simulink model "case2"  (R2024b)
settings: Solver=FixedStepAuto  StartTime=0  StopTime=1  FixedStep=1e-7  RelTol=1e-3
values from neighbouring files (symbols this model uses):
  SG_D_1_D = 0.01056    [IEEE9_case_parameters.m]    (also in case1_parameters.m; case2_parameters.m; case3_parameters.m; case4_parameters.m)
  SG_D_1_EnableSaturation = 0    [IEEE9_case_parameters.m]    (also in case1_parameters.m; case2_parameters.m; case3_parameters.m; case4_parameters.m)
  SG_D_1_f0 = 60    [IEEE9_case_parameters.m]    (also in case1_parameters.m; case2_parameters.m; case3_parameters.m; case4_parameters.m)
  SG_D_1_H = 7.5    [IEEE9_case_parameters.m]    (also in case1_parameters.m; case2_parameters.m; case3_parameters.m; case4_parameters.m)
  SG_D_1_K_A = 20    [IEEE9_case_parameters.m]    (also in case1_parameters.m; case2_parameters.m; case3_parameters.m; case4_parameters.m)
  SG_D_1_K_E = 1.000000e+1    (= 10)    [IEEE9_case_parameters.m]    (also in case1_parameters.m; case2_parameters.m; case3_parameters.m; case4_parameters.m)
  SG_D_1_K_F = 2.363    [IEEE9_case_parameters.m]    (also in case1_parameters.m; case2_parameters.m; case3_parameters.m; case4_parameters.m)
  SG_D_1_K_s = 0.5    [IEEE9_case_parameters.m]    (also in case1_parameters.m = 5; case2_parameters.m = 5; case3_parameters.m = 5; case4_parameters.m = 5)
  SG_D_1_R_a = 0.001088    [IEEE9_case_parameters.m]    (also in case1_parameters.m; case2_parameters.m; case3_parameters.m; case4_parameters.m)
  SG_D_1_S_A = 1    [IEEE9_case_parameters.m]    (also in case1_parameters.m; case2_parameters.m; case3_parameters.m; case4_parameters.m)
  SG_D_1_S_B = 0.103    [IEEE9_case_parameters.m]    (also in case1_parameters.m; case2_parameters.m; case3_parameters.m; case4_parameters.m)
  SG_D_1_S_N = 10.659857    [IEEE9_case_parameters.m]    (also in case1_parameters.m; case2_parameters.m; case3_parameters.m; case4_parameters.m)
  SG_D_1_SpeedPara = 200    [IEEE9_case_parameters.m]    (also in case1_parameters.m; case2_parameters.m; case3_parameters.m; case4_parameters.m)
  SG_D_1_T_0 = 0.720173    [IEEE9_case_parameters.m]    (also in case1_parameters.m = 0.755522; case2_parameters.m = 0.808931; case3_parameters.m = 0.869402; case4_parameters.m = 0.729316)
  SG_D_1_T_1 = 0.3    [IEEE9_case_parameters.m]    (also in case1_parameters.m; case2_parameters.m; case3_parameters.m; case4_parameters.m)
  SG_D_1_T_2 = 0.05    [IEEE9_case_parameters.m]    (also in case1_parameters.m; case2_parameters.m; case3_parameters.m; case4_parameters.m)
  SG_D_1_T_3 = 0.02    [IEEE9_case_parameters.m]    (also in case1_parameters.m; case2_parameters.m; case3_parameters.m; case4_parameters.m)
  SG_D_1_T_4 = 0.005    [IEEE9_case_parameters.m]    (also in case1_parameters.m; case2_parameters.m; case3_parameters.m; case4_parameters.m)
  SG_D_1_T_A = 0.02    [IEEE9_case_parameters.m]    (also in case1_parameters.m; case2_parameters.m; case3_parameters.m; case4_parameters.m)
  SG_D_1_T_dd = 8.000000e+0    (= 8)    [IEEE9_case_parameters.m]    (also in case1_parameters.m; case2_parameters.m; case3_parameters.m; case4_parameters.m)
  SG_D_1_T_ddd = 0.04    [IEEE9_case_parameters.m]    (also in case1_parameters.m; case2_parameters.m; case3_parameters.m; case4_parameters.m)
  SG_D_1_T_E = 0.314    [IEEE9_case_parameters.m]    (also in case1_parameters.m; case2_parameters.m; case3_parameters.m; case4_parameters.m)
  SG_D_1_T_F = 0.35    [IEEE9_case_parameters.m]    (also in case1_parameters.m; case2_parameters.m; case3_parameters.m; case4_parameters.m)
  SG_D_1_T_qd = 0.8    [IEEE9_case_parameters.m]    (also in case1_parameters.m; case2_parameters.m; case3_parameters.m; case4_parameters.m)
  SG_D_1_T_qdd = 0.02    [IEEE9_case_parameters.m]    (also in case1_parameters.m; case2_parameters.m; case3_parameters.m; case4_parameters.m)
  SG_D_1_T_speed = 0.1    [IEEE9_case_parameters.m]    (also in case1_parameters.m = 200; case2_parameters.m = 200; case3_parameters.m = 200; case4_parameters.m = 200)
  SG_D_1_T_w = 0.5    [IEEE9_case_parameters.m]    (also in case1_parameters.m; case2_parameters.m; case3_parameters.m; case4_parameters.m)
  SG_D_1_V_ref = 1.990276    [IEEE9_case_parameters.m]    (also in case1_parameters.m = 2.042296; case2_parameters.m = 2.051388; case3_parameters.m = 2.089584; case4_parameters.m = 2.01845)
  SG_D_1_w_ref = 376.991118    [IEEE9_case_parameters.m]    (also in case1_parameters.m; case2_parameters.m; case3_parameters.m; case4_parameters.m)
  SG_D_1_wb = 6.000000e+1    (= 60)    [IEEE9_case_parameters.m]    (also in case1_parameters.m; case2_parameters.m; case3_parameters.m; case4_parameters.m)
  SG_D_1_x_d = 1.9    [IEEE9_case_parameters.m]    (also in case1_parameters.m; case2_parameters.m; case3_parameters.m; case4_parameters.m)
  SG_D_1_x_dd = 0.302    [IEEE9_case_parameters.m]    (also in case1_parameters.m; case2_parameters.m; case3_parameters.m; case4_parameters.m)
  SG_D_1_x_ddd = 0.204    [IEEE9_case_parameters.m]    (also in case1_parameters.m; case2_parameters.m; case3_parameters.m; case4_parameters.m)
  SG_D_1_x_l = 0.05    [IEEE9_case_parameters.m]    (also in case1_parameters.m; case2_parameters.m; case3_parameters.m; case4_parameters.m)
  SG_D_1_x_q = 1.3    [IEEE9_case_parameters.m]    (also in case1_parameters.m; case2_parameters.m; case3_parameters.m; case4_parameters.m)
  SG_D_1_x_qd = 0.5    [IEEE9_case_parameters.m]    (also in case1_parameters.m; case2_parameters.m; case3_parameters.m; case4_parameters.m)
  SG_D_1_x_qdd = 0.3    [IEEE9_case_parameters.m]    (also in case1_parameters.m; case2_parameters.m; case3_parameters.m; case4_parameters.m)
  SG_D_2_D = 0.02    [IEEE9_case_parameters.m]    (also in case1_parameters.m; case2_parameters.m; case3_parameters.m; case4_parameters.m)
  SG_D_2_EnableSaturation = 0    [IEEE9_case_parameters.m]    (also in case1_parameters.m; case2_parameters.m; case3_parameters.m; case4_parameters.m)
  SG_D_2_f0 = 60    [IEEE9_case_parameters.m]    (also in case1_parameters.m; case2_parameters.m; case3_parameters.m; case4_parameters.m)
  SG_D_2_H = 8.000000e+0    (= 8)    [IEEE9_case_parameters.m]    (also in case1_parameters.m; case2_parameters.m; case3_parameters.m; case4_parameters.m)
  SG_D_2_K_A = 20    [IEEE9_case_parameters.m]    (also in case1_parameters.m; case2_parameters.m; case3_parameters.m; case4_parameters.m)
  SG_D_2_K_E = 1.000000e+1    (= 10)    [IEEE9_case_parameters.m]    (also in case1_parameters.m; case2_parameters.m; case3_parameters.m; case4_parameters.m)
  SG_D_2_K_F = 2.363    [IEEE9_case_parameters.m]    (also in case1_parameters.m; case2_parameters.m; case3_parameters.m; case4_parameters.m)
  SG_D_2_K_s = 0.5    [IEEE9_case_parameters.m]    (also in case1_parameters.m = 4; case2_parameters.m = 4; case3_parameters.m = 4; case4_parameters.m = 4)
  SG_D_2_R_a = 0.001088    [IEEE9_case_parameters.m]    (also in case1_parameters.m; case2_parameters.m; case3_parameters.m; case4_parameters.m)
  SG_D_2_S_A = 1    [IEEE9_case_parameters.m]    (also in case1_parameters.m; case2_parameters.m; case3_parameters.m; case4_parameters.m)
  SG_D_2_S_B = 0.103    [IEEE9_case_parameters.m]    (also in case1_parameters.m; case2_parameters.m; case3_parameters.m; case4_parameters.m)
  SG_D_2_S_N = 10.659857    [IEEE9_case_parameters.m]    (also in case1_parameters.m; case2_parameters.m; case3_parameters.m; case4_parameters.m)
  SG_D_2_SpeedPara = 200    [IEEE9_case_parameters.m]    (also in case1_parameters.m; case2_parameters.m; case3_parameters.m; case4_parameters.m)
  SG_D_2_T_0 = 1.632913    [IEEE9_case_parameters.m]    (also in case1_parameters.m = 1.632925; case2_parameters.m = 1.632915; case3_parameters.m = 1.632914; case4_parameters.m = 1.632927)
  SG_D_2_T_1 = 0.2    [IEEE9_case_parameters.m]    (also in case1_parameters.m; case2_parameters.m; case3_parameters.m; case4_parameters.m)
  SG_D_2_T_2 = 0.05    [IEEE9_case_parameters.m]    (also in case1_parameters.m; case2_parameters.m; case3_parameters.m; case4_parameters.m)
  SG_D_2_T_3 = 0.02    [IEEE9_case_parameters.m]    (also in case1_parameters.m; case2_parameters.m; case3_parameters.m; case4_parameters.m)
  SG_D_2_T_4 = 0.005    [IEEE9_case_parameters.m]    (also in case1_parameters.m; case2_parameters.m; case3_parameters.m; case4_parameters.m)
  SG_D_2_T_A = 0.02    [IEEE9_case_parameters.m]    (also in case1_parameters.m; case2_parameters.m; case3_parameters.m; case4_parameters.m)
  SG_D_2_T_dd = 7.9    [IEEE9_case_parameters.m]    (also in case1_parameters.m; case2_parameters.m; case3_parameters.m; case4_parameters.m)
  SG_D_2_T_ddd = 0.04    [IEEE9_case_parameters.m]    (also in case1_parameters.m; case2_parameters.m; case3_parameters.m; case4_parameters.m)
  SG_D_2_T_E = 0.314    [IEEE9_case_parameters.m]    (also in case1_parameters.m; case2_parameters.m; case3_parameters.m; case4_parameters.m)
  SG_D_2_T_F = 0.35    [IEEE9_case_parameters.m]    (also in case1_parameters.m; case2_parameters.m; case3_parameters.m; case4_parameters.m)
  SG_D_2_T_qd = 0.8    [IEEE9_case_parameters.m]    (also in case1_parameters.m; case2_parameters.m; case3_parameters.m; case4_parameters.m)
  SG_D_2_T_qdd = 0.015    [IEEE9_case_parameters.m]    (also in case1_parameters.m; case2_parameters.m; case3_parameters.m; case4_parameters.m)
  SG_D_2_T_speed = 0.1    [IEEE9_case_parameters.m]    (also in case1_parameters.m = 150; case2_parameters.m = 150; case3_parameters.m = 150; case4_parameters.m = 150)
  SG_D_2_T_w = 0.35    [IEEE9_case_parameters.m]    (also in case1_parameters.m; case2_parameters.m; case3_parameters.m; case4_parameters.m)
  SG_D_2_V_ref = 2.58547    [IEEE9_case_parameters.m]    (also in case1_parameters.m = 2.597896; case2_parameters.m = 2.587136; case3_parameters.m = 2.586042; case4_parameters.m = 2.599679)
  SG_D_2_w_ref = 376.991118    [IEEE9_case_parameters.m]    (also in case1_parameters.m; case2_parameters.m; case3_parameters.m; case4_parameters.m)
  SG_D_2_wb = 6.000000e+1    (= 60)    [IEEE9_case_parameters.m]    (also in case1_parameters.m; case2_parameters.m; case3_parameters.m; case4_parameters.m)
  SG_D_2_x_d = 1.8    [IEEE9_case_parameters.m]    (also in case1_parameters.m; case2_parameters.m; case3_parameters.m; case4_parameters.m)
  SG_D_2_x_dd = 0.302    [IEEE9_case_parameters.m]    (also in case1_parameters.m; case2_parameters.m; case3_parameters.m; case4_parameters.m)
  SG_D_2_x_ddd = 0.204    [IEEE9_case_parameters.m]    (also in case1_parameters.m; case2_parameters.m; case3_parameters.m; case4_parameters.m)
  SG_D_2_x_l = 0.05    [IEEE9_case_parameters.m]    (also in case1_parameters.m; case2_parameters.m; case3_parameters.m; case4_parameters.m)
  SG_D_2_x_q = 1.25    [IEEE9_case_parameters.m]    (also in case1_parameters.m; case2_parameters.m; case3_parameters.m; case4_parameters.m)
  SG_D_2_x_qd = 0.5    [IEEE9_case_parameters.m]    (also in case1_parameters.m; case2_parameters.m; case3_parameters.m; case4_parameters.m)
  SG_D_2_x_qdd = 0.3    [IEEE9_case_parameters.m]    (also in case1_parameters.m; case2_parameters.m; case3_parameters.m; case4_parameters.m)
  SG_D_3_D = 0.02    [IEEE9_case_parameters.m]    (also in case1_parameters.m; case2_parameters.m; case3_parameters.m; case4_parameters.m)
  SG_D_3_EnableSaturation = 0    [IEEE9_case_parameters.m]    (also in case1_parameters.m; case2_parameters.m; case3_parameters.m; case4_parameters.m)
  SG_D_3_f0 = 60    [IEEE9_case_parameters.m]    (also in case1_parameters.m; case2_parameters.m; case3_parameters.m; case4_parameters.m)
  SG_D_3_H = 7.7    [IEEE9_case_parameters.m]    (also in case1_parameters.m; case2_parameters.m; case3_parameters.m; case4_parameters.m)
  SG_D_3_K_A = 20    [IEEE9_case_parameters.m]    (also in case1_parameters.m; case2_parameters.m; case3_parameters.m; case4_parameters.m)
  SG_D_3_K_E = 1.000000e+1    (= 10)    [IEEE9_case_parameters.m]    (also in case1_parameters.m; case2_parameters.m; case3_parameters.m; case4_parameters.m)
  SG_D_3_K_F = 2.363    [IEEE9_case_parameters.m]    (also in case1_parameters.m; case2_parameters.m; case3_parameters.m; case4_parameters.m)
  SG_D_3_K_s = 0.2    [IEEE9_case_parameters.m]    (also in case1_parameters.m = 2; case2_parameters.m = 2; case3_parameters.m = 2; case4_parameters.m = 2)
  SG_D_3_R_a = 0.001088    [IEEE9_case_parameters.m]    (also in case1_parameters.m; case2_parameters.m; case3_parameters.m; case4_parameters.m)
  SG_D_3_S_A = 1    [IEEE9_case_parameters.m]    (also in case1_parameters.m; case2_parameters.m; case3_parameters.m; case4_parameters.m)
  SG_D_3_S_B = 0.103    [IEEE9_case_parameters.m]    (also in case1_parameters.m; case2_parameters.m; case3_parameters.m; case4_parameters.m)
  SG_D_3_S_N = 10.659857    [IEEE9_case_parameters.m]    (also in case1_parameters.m; case2_parameters.m; case3_parameters.m; case4_parameters.m)
  SG_D_3_SpeedPara = 200    [IEEE9_case_parameters.m]    (also in case1_parameters.m; case2_parameters.m; case3_parameters.m; case4_parameters.m)
  SG_D_3_T_0 = 0.850788    [IEEE9_case_parameters.m]    (also in case1_parameters.m = 0.850786; case2_parameters.m = 0.850787; case3_parameters.m; case4_parameters.m = 0.850786)
  SG_D_3_T_1 = 0.2    [IEEE9_case_parameters.m]    (also in case1_parameters.m; case2_parameters.m; case3_parameters.m; case4_parameters.m)
  SG_D_3_T_2 = 0.05    [IEEE9_case_parameters.m]    (also in case1_parameters.m; case2_parameters.m; case3_parameters.m; case4_parameters.m)
  SG_D_3_T_3 = 0.02    [IEEE9_case_parameters.m]    (also in case1_parameters.m; case2_parameters.m; case3_parameters.m; case4_parameters.m)
  SG_D_3_T_4 = 0.005    [IEEE9_case_parameters.m]    (also in case1_parameters.m; case2_parameters.m; case3_parameters.m; case4_parameters.m)
  SG_D_3_T_A = 0.02    [IEEE9_case_parameters.m]    (also in case1_parameters.m; case2_parameters.m; case3_parameters.m; case4_parameters.m)
  SG_D_3_T_dd = 8.1    [IEEE9_case_parameters.m]    (also in case1_parameters.m; case2_parameters.m; case3_parameters.m; case4_parameters.m)
  SG_D_3_T_ddd = 0.04    [IEEE9_case_parameters.m]    (also in case1_parameters.m; case2_parameters.m; case3_parameters.m; case4_parameters.m)
  SG_D_3_T_E = 0.314    [IEEE9_case_parameters.m]    (also in case1_parameters.m; case2_parameters.m; case3_parameters.m; case4_parameters.m)
  SG_D_3_T_F = 0.35    [IEEE9_case_parameters.m]    (also in case1_parameters.m; case2_parameters.m; case3_parameters.m; case4_parameters.m)
  SG_D_3_T_qd = 0.8    [IEEE9_case_parameters.m]    (also in case1_parameters.m; case2_parameters.m; case3_parameters.m; case4_parameters.m)
  SG_D_3_T_qdd = 0.015    [IEEE9_case_parameters.m]    (also in case1_parameters.m; case2_parameters.m; case3_parameters.m; case4_parameters.m)
  SG_D_3_T_speed = 0.1    [IEEE9_case_parameters.m]    (also in case1_parameters.m = 180; case2_parameters.m = 180; case3_parameters.m = 180; case4_parameters.m = 180)
  SG_D_3_T_w = 0.4    [IEEE9_case_parameters.m]    (also in case1_parameters.m; case2_parameters.m; case3_parameters.m; case4_parameters.m)
  SG_D_3_V_ref = 1.892727    [IEEE9_case_parameters.m]    (also in case1_parameters.m = 1.906439; case2_parameters.m = 1.895535; case3_parameters.m = 1.892105; case4_parameters.m = 1.906598)
  SG_D_3_w_ref = 376.991118    [IEEE9_case_parameters.m]    (also in case1_parameters.m; case2_parameters.m; case3_parameters.m; case4_parameters.m)
  SG_D_3_wb = 6.000000e+1    (= 60)    [IEEE9_case_parameters.m]    (also in case1_parameters.m; case2_parameters.m; case3_parameters.m; case4_parameters.m)
  SG_D_3_x_d = 1.85    [IEEE9_case_parameters.m]    (also in case1_parameters.m; case2_parameters.m; case3_parameters.m; case4_parameters.m)
  SG_D_3_x_dd = 0.302    [IEEE9_case_parameters.m]    (also in case1_parameters.m; case2_parameters.m; case3_parameters.m; case4_parameters.m)
  SG_D_3_x_ddd = 0.204    [IEEE9_case_parameters.m]    (also in case1_parameters.m; case2_parameters.m; case3_parameters.m; case4_parameters.m)
  SG_D_3_x_l = 0.05    [IEEE9_case_parameters.m]    (also in case1_parameters.m; case2_parameters.m; case3_parameters.m; case4_parameters.m)
  SG_D_3_x_q = 1.2    [IEEE9_case_parameters.m]    (also in case1_parameters.m; case2_parameters.m; case3_parameters.m; case4_parameters.m)
  SG_D_3_x_qd = 0.5    [IEEE9_case_parameters.m]    (also in case1_parameters.m; case2_parameters.m; case3_parameters.m; case4_parameters.m)
  SG_D_3_x_qdd = 0.3    [IEEE9_case_parameters.m]    (also in case1_parameters.m; case2_parameters.m; case3_parameters.m; case4_parameters.m)
(part 11 of 12)

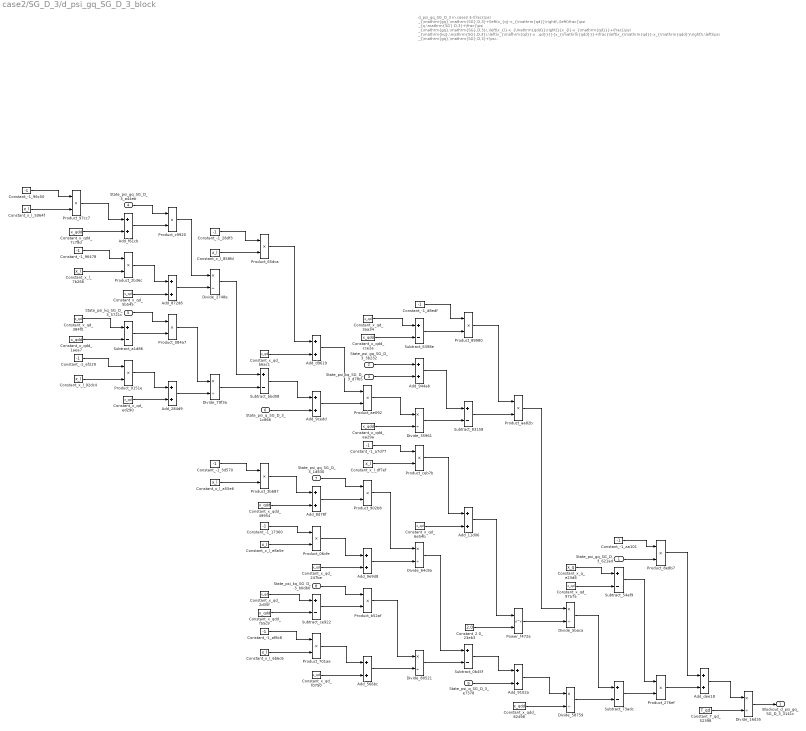
== system case2/SG_D_3/d_psi_gq_SG_D_3_block ==
  note: d_psi_gq_SG_D_3 in case2
      | $-\frac{\psi _{\mathrm{gq},\mathrm{SG},D,3}+\left(x_{q}-x_{\mathrm{qd}}\right)\,\left(\frac{\psi _{q,\mathrm{SG},D,3}+\frac{\psi _{\mathrm{gq},\mathrm{SG},D,3}\,\left(x_{l}-x_{\mathrm{qdd}}\right)}{x_{l}-x_{\mathrm{qd}}}+\frac{\psi _{\mathrm{kq},\mathrm{SG},D,3}\,\left(x_{\mathrm{qd}}-x_{\mathrm{qdd}}\right)}{x_{l}-x_{\mathrm{qd}}}}{x_{\mathrm{qdd}}}+\frac{\left(x_{\mathrm{qd}}-x_{\mathrm{qdd}}\right)\,\left(\psi _{\mathrm{gq},\mathrm{SG},D,3}+\psi _{\mathrm{kq},\mathrm{SG},D,3}+\frac{\left(x_{l}-x_{\mathrm{qd}}\right)\,\left(\psi _{q,\mathrm{SG},D,3}+\frac{\psi _{\mathrm{gq},\mathrm{SG},D,3}\,\left(x_{l}-x_{\mathrm{qdd}}\right)}{x_{l}-x_{\mathrm{qd}}}+\frac{\psi _{\mathrm{kq},\mathrm{SG},D,3}\,\left(x_{\mathrm{qd}}-x_{\mathrm{qdd}}\right)}{x_{l}-x_{\mathrm{qd}}}\right)}{x_{\mathrm{qdd}}}\right)}{{\left(x_{l}-x_{\mathrm{qd}}\right)}^2}\right)}{T_{\mathrm{qd}}}$
      | Automatically generated on 2025-10-31 18:55:42 .
  State_psi_gq_SG_D_3_621ad : Inport
  State_psi_gq_SG_D_3_3b232 : Inport  Port=2
  State_psi_kq_SG_D_3_d7fb5 : Inport  Port=3
  State_psi_gq_SG_D_3_a44eb : Inport  Port=4
  State_psi_kq_SG_D_3_5721c : Inport  Port=5
  State_psi_q_SG_D_3_1c866 : Inport  Port=6
  State_psi_gq_SG_D_3_1d830 : Inport  Port=7
  State_psi_kq_SG_D_3_b0db0 : Inport  Port=8
  State_psi_q_SG_D_3_e7378 : Inport  Port=9
  Add_11d06 : Sum
  Add_284d9 : Sum
  Add_566bc : Sum
  Add_872d8 : Sum
  Add_8d78f : Sum
  Add_9102a : Sum
  Add_944ab : Sum
  Add_9cedd : Sum
  Add_9e9d8 : Sum
  Add_d9619 : Sum
  Add_dee18 : Sum
  Add_f61cb : Sum
  Constant_-1_17360 : Constant  Value=-1
  Constant_-1_28df3 : Constant  Value=-1
  Constant_-1_3d570 : Constant  Value=-1
  Constant_-1_96478 : Constant  Value=-1
  Constant_-1_96c50 : Constant  Value=-1
  Constant_-1_a7d77 : Constant  Value=-1
  Constant_-1_aa101 : Constant  Value=-1
  Constant_-1_af8c8 : Constant  Value=-1
  Constant_-1_d8edf : Constant  Value=-1
  Constant_-1_ef229 : Constant  Value=-1
  Constant_2.0_23eb3 : Constant  Value=2.0
  Constant_T_qd_52398 : Constant  Value=T_qd
  Constant_x_l_5064f : Constant  Value=x_l
  Constant_x_l_6b6c6 : Constant  Value=x_l
  Constant_x_l_7b266 : Constant  Value=x_l
  Constant_x_l_858fd : Constant  Value=x_l
  Constant_x_l_92dc4 : Constant  Value=x_l
  Constant_x_l_a55e6 : Constant  Value=x_l
  Constant_x_l_df7ef : Constant  Value=x_l
  Constant_x_l_e8a5e : Constant  Value=x_l
  Constant_x_q_e23d8 : Constant  Value=x_q
  Constant_x_qd_247be : Constant  Value=x_qd
  Constant_x_qd_2d35f : Constant  Value=x_qd
  Constant_x_qd_384f0 : Constant  Value=x_qd
  Constant_x_qd_3aa34 : Constant  Value=x_qd
  Constant_x_qd_5b545 : Constant  Value=x_qd
  Constant_x_qd_6e54b : Constant  Value=x_qd
  Constant_x_qd_97a7a : Constant  Value=x_qd
  Constant_x_qd_b6ac1 : Constant  Value=x_qd
  Constant_x_qd_ed290 : Constant  Value=x_qd
  Constant_x_qd_f0750 : Constant  Value=x_qd
  Constant_x_qdd_1aea7 : Constant  Value=x_qdd
  Constant_x_qdd_49954 : Constant  Value=x_qdd
  Constant_x_qdd_7c78d : Constant  Value=x_qdd
  Constant_x_qdd_82498 : Constant  Value=x_qdd
  Constant_x_qdd_cce2a : Constant  Value=x_qdd
  Constant_x_qdd_ea29a : Constant  Value=x_qdd
  Constant_x_qdd_f55c9 : Constant  Value=x_qdd
  Divide_16d35 : Product  Inputs=*/
  Divide_2748e : Product  Inputs=*/
  Divide_35961 : Product  Inputs=*/
  Divide_58759 : Product  Inputs=*/
  Divide_5baca : Product  Inputs=*/
  Divide_64c8a : Product  Inputs=*/
  Divide_79f3a : Product  Inputs=*/
  Divide_80521 : Product  Inputs=*/
  Power_f472a : Math  Operator=pow
  Product_0151e : Product
  Product_06cfe : Product
  Product_084a7 : Product
  Product_276ef : Product
  Product_2b36c : Product
  Product_3b687 : Product
  Product_65dca : Product
  Product_701ae : Product
  Product_89980 : Product
  Product_8e8b7 : Product
  Product_902b8 : Product
  Product_97cc7 : Product
  Product_aa82b : Product
  Product_ae092 : Product
  Product_b52af : Product
  Product_c9920 : Product
  Product_ceb7b : Product
  Subtract_0b45f : Sum  Inputs=+-
  Subtract_54af9 : Sum  Inputs=+-
  Subtract_6398e : Sum  Inputs=+-
  Subtract_73adc : Sum  Inputs=+-
  Subtract_83158 : Sum  Inputs=+-
  Subtract_a1d86 : Sum  Inputs=+-
  Subtract_bbd08 : Sum  Inputs=+-
  Subtract_ce922 : Sum  Inputs=+-
  Blockout_d_psi_gq_SG_D_3_3141c : Outport
  wires:
  Constant_x_l_df7ef/1 -> Product_ceb7b/2
  Constant_x_qd_384f0/1 -> Subtract_a1d86/1
  Add_d9619/1 -> Product_ae092/1
  Constant_-1_96c50/1 -> Product_97cc7/1
  Add_f61cb/1 -> Product_c9920/2
  Constant_x_qdd_1aea7/1 -> Subtract_a1d86/2
  Constant_x_qd_b6ac1/1 -> Add_d9619/2
  Constant_x_l_5064f/1 -> Product_97cc7/2
  Constant_x_l_7b266/1 -> Product_2b36c/2
  Add_566bc/1 -> Divide_80521/2
  State_psi_kq_SG_D_3_d7fb5/1 -> Add_944ab/2
  Constant_x_qdd_7c78d/1 -> Add_f61cb/2
  Product_97cc7/1 -> Add_f61cb/1
  Constant_x_qd_f0750/1 -> Add_566bc/2
  Product_89980/1 -> Product_aa82b/1
  Constant_-1_3d570/1 -> Product_3b687/1
  Constant_-1_96478/1 -> Product_2b36c/1
  Constant_-1_ef229/1 -> Product_0151e/1
  Constant_x_l_92dc4/1 -> Product_0151e/2
  Constant_-1_d8edf/1 -> Product_89980/1
  Constant_-1_aa101/1 -> Product_8e8b7/1
  State_psi_gq_SG_D_3_a44eb/1 -> Product_c9920/1
  Product_3b687/1 -> Add_8d78f/1
  Product_2b36c/1 -> Add_872d8/1
  Product_701ae/1 -> Add_566bc/1
  Constant_x_qd_5b545/1 -> Add_872d8/2
  Constant_-1_17360/1 -> Product_06cfe/1
  State_psi_kq_SG_D_3_5721c/1 -> Product_084a7/1
  Subtract_a1d86/1 -> Product_084a7/2
  Product_0151e/1 -> Add_284d9/1
  Add_8d78f/1 -> Product_902b8/2
  Add_872d8/1 -> Divide_2748e/2
  Constant_x_qd_ed290/1 -> Add_284d9/2
  Product_c9920/1 -> Divide_2748e/1
  Constant_T_qd_52398/1 -> Divide_16d35/2
  Product_06cfe/1 -> Add_9e9d8/1
  Product_084a7/1 -> Divide_79f3a/1
  Product_b52af/1 -> Divide_80521/1
  Add_284d9/1 -> Divide_79f3a/2
  Constant_-1_28df3/1 -> Product_65dca/1
  Constant_x_qdd_ea29a/1 -> Divide_35961/2
  Constant_x_l_858fd/1 -> Product_65dca/2
  Divide_2748e/1 -> Subtract_bbd08/1
  Constant_x_qd_97a7a/1 -> Subtract_54af9/2
  Add_9e9d8/1 -> Divide_64c8a/2
  Divide_79f3a/1 -> Subtract_bbd08/2
  Constant_x_l_a55e6/1 -> Product_3b687/2
  Product_65dca/1 -> Add_d9619/1
  Constant_-1_a7d77/1 -> Product_ceb7b/1
  Constant_x_l_e8a5e/1 -> Product_06cfe/2
  Subtract_bbd08/1 -> Add_9cedd/1
  State_psi_q_SG_D_3_1c866/1 -> Add_9cedd/2
  Constant_-1_af8c8/1 -> Product_701ae/1
  Constant_x_qdd_49954/1 -> Add_8d78f/2
  Constant_x_qd_2d35f/1 -> Subtract_ce922/1
  Constant_x_qdd_f55c9/1 -> Subtract_ce922/2
  Constant_x_l_6b6c6/1 -> Product_701ae/2
  Add_9cedd/1 -> Product_ae092/2
  Constant_x_qdd_cce2a/1 -> Subtract_6398e/2
  State_psi_gq_SG_D_3_1d830/1 -> Product_902b8/1
  Constant_x_qd_247be/1 -> Add_9e9d8/2
  Divide_5baca/1 -> Subtract_73adc/1
  State_psi_kq_SG_D_3_b0db0/1 -> Product_b52af/1
  Subtract_ce922/1 -> Product_b52af/2
  Constant_x_qd_3aa34/1 -> Subtract_6398e/1
  State_psi_gq_SG_D_3_3b232/1 -> Add_944ab/1
  Product_ae092/1 -> Divide_35961/1
  Product_902b8/1 -> Divide_64c8a/1
  Subtract_6398e/1 -> Product_89980/2
  Add_944ab/1 -> Subtract_83158/1
  Divide_35961/1 -> Subtract_83158/2
  Product_ceb7b/1 -> Add_11d06/1
  Constant_x_qd_6e54b/1 -> Add_11d06/2
  Divide_64c8a/1 -> Subtract_0b45f/1
  Divide_80521/1 -> Subtract_0b45f/2
  Subtract_83158/1 -> Product_aa82b/2
  Add_11d06/1 -> Power_f472a/1
  Constant_2.0_23eb3/1 -> Power_f472a/2
  Subtract_0b45f/1 -> Add_9102a/1
  State_psi_q_SG_D_3_e7378/1 -> Add_9102a/2
  Product_aa82b/1 -> Divide_5baca/1
  Power_f472a/1 -> Divide_5baca/2
  Add_9102a/1 -> Divide_58759/1
  Constant_x_qdd_82498/1 -> Divide_58759/2
  Constant_x_q_e23d8/1 -> Subtract_54af9/1
  Divide_58759/1 -> Subtract_73adc/2
  State_psi_gq_SG_D_3_621ad/1 -> Product_8e8b7/2
  Subtract_54af9/1 -> Product_276ef/1
  Subtract_73adc/1 -> Product_276ef/2
  Product_8e8b7/1 -> Add_dee18/1
  Product_276ef/1 -> Add_dee18/2
  Add_dee18/1 -> Divide_16d35/1
  Divide_16d35/1 -> Blockout_d_psi_gq_SG_D_3_3141c/1

== system case2/SG_D_3/d_psi_kq_SG_D_3_block ==
  note: d_psi_kq_SG_D_3 in case2
      | $-\frac{\psi _{\mathrm{gq},\mathrm{SG},D,3}+\psi _{\mathrm{kq},\mathrm{SG},D,3}+\frac{\left(x_{l}-x_{\mathrm{qd}}\right)\,\left(\psi _{q,\mathrm{SG},D,3}+\frac{\psi _{\mathrm{gq},\mathrm{SG},D,3}\,\left(x_{l}-x_{\mathrm{qdd}}\right)}{x_{l}-x_{\mathrm{qd}}}+\frac{\psi _{\mathrm{kq},\mathrm{SG},D,3}\,\left(x_{\mathrm{qd}}-x_{\mathrm{qdd}}\right)}{x_{l}-x_{\mathrm{qd}}}\right)}{x_{\mathrm{qdd}}}}{T_{\mathrm{qdd}}}$
      | Automatically generated on 2025-10-31 18:55:45 .
  State_psi_gq_SG_D_3_a1641 : Inport
  State_psi_kq_SG_D_3_4633d : Inport  Port=2
  State_psi_gq_SG_D_3_25fe6 : Inport  Port=3
  State_psi_kq_SG_D_3_8378f : Inport  Port=4
  State_psi_q_SG_D_3_91d06 : Inport  Port=5
  Add_0913b : Sum
  Add_0e2f8 : Sum
  Add_1463d : Sum
  Add_5b1aa : Sum
  Add_98ac4 : Sum
  Add_f6f6b : Sum
  Constant_-1_18cc8 : Constant  Value=-1
  Constant_-1_671a6 : Constant  Value=-1
  Constant_-1_9164e : Constant  Value=-1
  Constant_-1_b214a : Constant  Value=-1
  Constant_-1_b9c1f : Constant  Value=-1
  Constant_T_qdd_fa348 : Constant  Value=T_qdd
  Constant_x_l_0d720 : Constant  Value=x_l
  Constant_x_l_27bc0 : Constant  Value=x_l
  Constant_x_l_9d6f4 : Constant  Value=x_l
  Constant_x_l_eeec5 : Constant  Value=x_l
  Constant_x_qd_81bcb : Constant  Value=x_qd
  Constant_x_qd_8576b : Constant  Value=x_qd
  Constant_x_qd_ce903 : Constant  Value=x_qd
  Constant_x_qd_d482d : Constant  Value=x_qd
  Constant_x_qdd_1a115 : Constant  Value=x_qdd
  Constant_x_qdd_b4830 : Constant  Value=x_qdd
  Constant_x_qdd_be369 : Constant  Value=x_qdd
  Divide_586cf : Product  Inputs=*/
  Divide_61cd8 : Product  Inputs=*/
  Divide_82a36 : Product  Inputs=*/
  Divide_87941 : Product  Inputs=*/
  Product_0f59d : Product
  Product_51f52 : Product
  Product_5c108 : Product
  Product_95a58 : Product
  Product_d62af : Product
  Product_dc04a : Product
  Product_e139f : Product
  Product_e2346 : Product
  Subtract_1e6f8 : Sum  Inputs=+-
  Subtract_d01a1 : Sum  Inputs=+-
  Subtract_dbf3a : Sum  Inputs=+-
  Blockout_d_psi_kq_SG_D_3_c5bf2 : Outport
  wires:
  State_psi_q_SG_D_3_91d06/1 -> Add_f6f6b/2
  Constant_-1_b214a/1 -> Product_e2346/1
  Constant_-1_18cc8/1 -> Product_e139f/1
  Constant_-1_671a6/1 -> Product_d62af/1
  Constant_x_l_27bc0/1 -> Product_e2346/2
  Constant_x_qdd_b4830/1 -> Add_0e2f8/2
  Product_5c108/1 -> Add_1463d/1
  Constant_x_l_0d720/1 -> Product_e139f/2
  Constant_x_qd_ce903/1 -> Subtract_dbf3a/1
  Product_e139f/1 -> Add_0e2f8/1
  Constant_x_l_9d6f4/1 -> Product_dc04a/2
  Constant_x_qdd_be369/1 -> Subtract_dbf3a/2
  Constant_-1_9164e/1 -> Product_5c108/1
  Constant_x_l_eeec5/1 -> Product_5c108/2
  State_psi_gq_SG_D_3_25fe6/1 -> Product_0f59d/1
  Add_0e2f8/1 -> Product_0f59d/2
  Add_f6f6b/1 -> Product_95a58/2
  Product_e2346/1 -> Add_5b1aa/1
  Constant_x_qd_d482d/1 -> Add_5b1aa/2
  State_psi_kq_SG_D_3_8378f/1 -> Product_51f52/1
  Subtract_dbf3a/1 -> Product_51f52/2
  Add_5b1aa/1 -> Divide_82a36/2
  Constant_x_qd_8576b/1 -> Add_1463d/2
  Product_0f59d/1 -> Divide_82a36/1
  Product_51f52/1 -> Divide_61cd8/1
  Add_1463d/1 -> Divide_61cd8/2
  Constant_-1_b9c1f/1 -> Product_dc04a/1
  Divide_82a36/1 -> Subtract_1e6f8/1
  Add_0913b/1 -> Divide_586cf/1
  Divide_61cd8/1 -> Subtract_1e6f8/2
  Divide_586cf/1 -> Blockout_d_psi_kq_SG_D_3_c5bf2/1
  Product_dc04a/1 -> Add_98ac4/1
  Constant_x_qd_81bcb/1 -> Add_98ac4/2
  Subtract_1e6f8/1 -> Add_f6f6b/1
  State_psi_gq_SG_D_3_a1641/1 -> Product_d62af/2
  Add_98ac4/1 -> Product_95a58/1
  Constant_T_qdd_fa348/1 -> Divide_586cf/2
  Product_d62af/1 -> Subtract_d01a1/1
  State_psi_kq_SG_D_3_4633d/1 -> Subtract_d01a1/2
  Product_95a58/1 -> Divide_87941/1
  Constant_x_qdd_1a115/1 -> Divide_87941/2
  Subtract_d01a1/1 -> Add_0913b/1
  Divide_87941/1 -> Add_0913b/2

== system case2/SG_D_3/d_psi_q_SG_D_3_block ==
  note: d_psi_q_SG_D_3 in case2
      | $2\,\pi \,f_{0}\,\left(v_{d,\mathrm{SG},D,3}\,\cos\left(\theta _{\mathrm{SG},D,3}\right)+v_{q,\mathrm{SG},D,3}\,\sin\left(\theta _{\mathrm{SG},D,3}\right)-\frac{R_{a}\,\left(\psi _{q,\mathrm{SG},D,3}+\frac{\psi _{\mathrm{gq},\mathrm{SG},D,3}\,\left(x_{l}-x_{\mathrm{qdd}}\right)}{x_{l}-x_{\mathrm{qd}}}+\frac{\psi _{\mathrm{kq},\mathrm{SG},D,3}\,\left(x_{\mathrm{qd}}-x_{\mathrm{qdd}}\right)}{x_{l}-x_{\mathrm{qd}}}\right)}{x_{\mathrm{qdd}}}-\frac{\psi _{d,\mathrm{SG},D,3}\,w_{\mathrm{SG},D,3}}{2\,f_{0}\,\pi }\right)$
      | Automatically generated on 2025-10-31 18:55:28 .
  State_psi_gq_SG_D_3_520bc : Inport
  State_psi_kq_SG_D_3_0e323 : Inport  Port=2
  State_psi_q_SG_D_3_df188 : Inport  Port=3
  Input_v_d_SG_D_3_18c9f : Inport  Port=4
  State_theta_SG_D_3_06d3e : Inport  Port=5
  Input_v_q_SG_D_3_33c03 : Inport  Port=6
  State_theta_SG_D_3_49b48 : Inport  Port=7
  State_psi_d_SG_D_3_6d66b : Inport  Port=8
  State_w_SG_D_3_6302a : Inport  Port=9
  Add_1a9c2 : Sum
  Add_1c02a : Sum
  Add_49d1b : Sum
  Add_5f7bb : Sum
  Add_78865 : Sum
  Constant_-1_128b7 : Constant  Value=-1
  Constant_-1_7ec3f : Constant  Value=-1
  Constant_-1_b7099 : Constant  Value=-1
  Constant_-2.0_efa81 : Constant  Value=-2.0
  Constant_2.0_5ef24 : Constant  Value=2.0
  Constant_R_a_11599 : Constant  Value=R_a
  Constant_f0_8dcae : Constant  Value=f0
  Constant_f0_a0bb5 : Constant  Value=f0
  Constant_pi_629cf : Constant  Value=pi
  Constant_pi_b321e : Constant  Value=pi
  Constant_x_l_4fa8b : Constant  Value=x_l
  Constant_x_l_78e36 : Constant  Value=x_l
  Constant_x_l_e6a60 : Constant  Value=x_l
  Constant_x_qd_51269 : Constant  Value=x_qd
  Constant_x_qd_88603 : Constant  Value=x_qd
  Constant_x_qd_e1e05 : Constant  Value=x_qd
  Constant_x_qdd_dc628 : Constant  Value=x_qdd
  Constant_x_qdd_f8aa7 : Constant  Value=x_qdd
  Constant_x_qdd_ffffd : Constant  Value=x_qdd
  Divide_014c6 : Product  Inputs=*/
  Divide_5baae : Product  Inputs=*/
  Divide_f78e2 : Product  Inputs=*/
  Divide_ffb84 : Product  Inputs=*/
  MathFunc_cos_2cd5b : Trigonometry  Operator=cos
  MathFunc_sin_bdfb3 : Trigonometry
  Product_0d7e3 : Product
  Product_1e447 : Product
  Product_3d7ca : Product
  Product_5ff76 : Product
  Product_63c68 : Product
  Product_65b03 : Product
  Product_70f78 : Product
  Product_83c96 : Product
  Product_8467a : Product
  Product_87f7a : Product
  Product_964bc : Product
  Product_ab8a9 : Product
  Product_e3438 : Product
  Product_ebb0d : Product
  Subtract_25259 : Sum  Inputs=+-
  Subtract_74f0f : Sum  Inputs=+-
  Subtract_8e9b0 : Sum  Inputs=+-
  Subtract_fb89c : Sum  Inputs=+-
  Blockout_d_psi_q_SG_D_3_0049f : Outport
  wires:
  Constant_x_qd_e1e05/1 -> Subtract_25259/1
  Constant_pi_629cf/1 -> Product_3d7ca/2
  Product_0d7e3/1 -> Divide_014c6/1
  Constant_x_l_4fa8b/1 -> Product_63c68/2
  Constant_f0_a0bb5/1 -> Product_ebb0d/2
  State_w_SG_D_3_6302a/1 -> Product_1e447/2
  Constant_-1_7ec3f/1 -> Product_964bc/1
  Constant_x_qdd_dc628/1 -> Add_1c02a/2
  Input_v_d_SG_D_3_18c9f/1 -> Product_87f7a/1
  Constant_x_qdd_ffffd/1 -> Subtract_25259/2
  Constant_x_l_e6a60/1 -> Product_964bc/2
  Divide_f78e2/1 -> Add_49d1b/2
  Product_964bc/1 -> Add_1c02a/1
  Constant_2.0_5ef24/1 -> Product_3d7ca/1
  Add_78865/1 -> Product_0d7e3/2
  Constant_-1_128b7/1 -> Product_63c68/1
  Constant_x_qd_88603/1 -> Add_1a9c2/2
  Constant_-1_b7099/1 -> Product_ab8a9/1
  Subtract_fb89c/1 -> Subtract_8e9b0/1
  Constant_x_l_78e36/1 -> Product_ab8a9/2
  Subtract_8e9b0/1 -> Add_49d1b/1
  Constant_f0_8dcae/1 -> Product_65b03/2
  State_theta_SG_D_3_49b48/1 -> MathFunc_sin_bdfb3/1
  Constant_x_qd_51269/1 -> Add_5f7bb/2
  State_psi_gq_SG_D_3_520bc/1 -> Product_5ff76/1
  Add_1c02a/1 -> Product_5ff76/2
  Product_3d7ca/1 -> Product_65b03/1
  Product_63c68/1 -> Add_5f7bb/1
  State_psi_kq_SG_D_3_0e323/1 -> Product_8467a/1
  Subtract_25259/1 -> Product_8467a/2
  Product_ab8a9/1 -> Add_1a9c2/1
  MathFunc_sin_bdfb3/1 -> Product_83c96/2
  Product_5ff76/1 -> Divide_5baae/1
  Product_65b03/1 -> Divide_f78e2/2
  Add_5f7bb/1 -> Divide_5baae/2
  Product_8467a/1 -> Divide_ffb84/1
  Add_1a9c2/1 -> Divide_ffb84/2
  Input_v_q_SG_D_3_33c03/1 -> Product_83c96/1
  Divide_5baae/1 -> Subtract_74f0f/1
  Subtract_74f0f/1 -> Add_78865/1
  Divide_ffb84/1 -> Subtract_74f0f/2
  Divide_014c6/1 -> Subtract_fb89c/1
  State_psi_q_SG_D_3_df188/1 -> Add_78865/2
  Product_83c96/1 -> Subtract_8e9b0/2
  Constant_R_a_11599/1 -> Product_0d7e3/1
  State_theta_SG_D_3_06d3e/1 -> MathFunc_cos_2cd5b/1
  Constant_x_qdd_f8aa7/1 -> Divide_014c6/2
  MathFunc_cos_2cd5b/1 -> Product_87f7a/2
  Constant_-2.0_efa81/1 -> Product_e3438/1
  Product_87f7a/1 -> Subtract_fb89c/2
  State_psi_d_SG_D_3_6d66b/1 -> Product_1e447/1
  Constant_pi_b321e/1 -> Product_e3438/2
  Product_1e447/1 -> Divide_f78e2/1
  Product_e3438/1 -> Product_ebb0d/1
  Product_ebb0d/1 -> Product_70f78/1
  Add_49d1b/1 -> Product_70f78/2
  Product_70f78/1 -> Blockout_d_psi_q_SG_D_3_0049f/1

== system case2/SG_D_3/d_theta_SG_D_3_block ==
  note: d_theta_SG_D_3 in case2
      | $w_{\mathrm{SG},D,3}-2\,\pi \,f_{0}$
      | Automatically generated on 2025-10-31 18:55:53 .
  State_w_SG_D_3_3d54c : Inport
  Add_acd9b : Sum
  Constant_-2.0_95b18 : Constant  Value=-2.0
  Constant_f0_1e811 : Constant  Value=f0
  Constant_pi_f9e96 : Constant  Value=pi
  Product_8b2b7 : Product
  Product_b6d83 : Product
  Blockout_d_theta_SG_D_3_7f2c9 : Outport
  wires:
  Constant_-2.0_95b18/1 -> Product_8b2b7/1
  Constant_pi_f9e96/1 -> Product_8b2b7/2
  State_w_SG_D_3_3d54c/1 -> Add_acd9b/2
  Product_8b2b7/1 -> Product_b6d83/1
  Constant_f0_1e811/1 -> Product_b6d83/2
  Product_b6d83/1 -> Add_acd9b/1
  Add_acd9b/1 -> Blockout_d_theta_SG_D_3_7f2c9/1

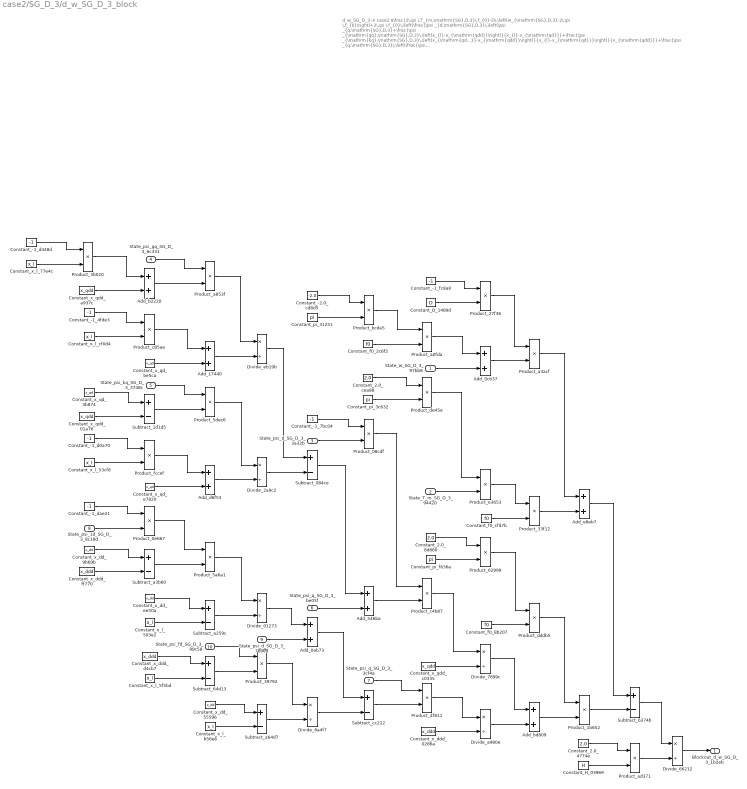
== system case2/SG_D_3/d_w_SG_D_3_block ==
  note: d_w_SG_D_3 in case2
      | $\frac{2\,\pi \,T_{m,\mathrm{SG},D,3}\,f_{0}-D\,\left(w_{\mathrm{SG},D,3}-2\,\pi \,f_{0}\right)+2\,\pi \,f_{0}\,\left(\frac{\psi _{d,\mathrm{SG},D,3}\,\left(\psi _{q,\mathrm{SG},D,3}+\frac{\psi _{\mathrm{gq},\mathrm{SG},D,3}\,\left(x_{l}-x_{\mathrm{qdd}}\right)}{x_{l}-x_{\mathrm{qd}}}+\frac{\psi _{\mathrm{kq},\mathrm{SG},D,3}\,\left(x_{\mathrm{qd}}-x_{\mathrm{qdd}}\right)}{x_{l}-x_{\mathrm{qd}}}\right)}{x_{\mathrm{qdd}}}+\frac{\psi _{q,\mathrm{SG},D,3}\,\left(\frac{\psi _{\mathrm{1d},\mathrm{SG},D,3}\,\left(x_{\mathrm{dd}}-x_{\mathrm{ddd}}\right)}{x_{\mathrm{dd}}-x_{l}}-\psi _{d,\mathrm{SG},D,3}+\frac{\psi _{\mathrm{fd},\mathrm{SG},D,3}\,\left(x_{\mathrm{ddd}}-x_{l}\right)}{x_{\mathrm{dd}}-x_{l}}\right)}{x_{\mathrm{ddd}}}\right)}{2\,H}$
      | Automatically generated on 2025-10-31 18:55:51 .
  State_w_SG_D_3_97bb8 : Inport
  State_T_m_SG_D_3_94420 : Inport  Port=2
  State_psi_d_SG_D_3_3a32b : Inport  Port=3
  State_psi_gq_SG_D_3_6c331 : Inport  Port=4
  State_psi_kq_SG_D_3_3748c : Inport  Port=5
  State_psi_q_SG_D_3_be05f : Inport  Port=6
  State_psi_q_SG_D_3_3cf4a : Inport  Port=7
  State_psi_1d_SG_D_3_8c18d : Inport  Port=8
  State_psi_d_SG_D_3_7b9ed : Inport  Port=9
  State_psi_fd_SG_D_3_99c58 : Inport  Port=10
  Add_0ab73 : Sum
  Add_0cb37 : Sum
  Add_17440 : Sum
  Add_546ba : Sum
  Add_b2220 : Sum
  Add_bd809 : Sum
  Add_d6f53 : Sum
  Add_e8eb7 : Sum
  Constant_-1_4fde3 : Constant  Value=-1
  Constant_-1_7bc04 : Constant  Value=-1
  Constant_-1_d0a70 : Constant  Value=-1
  Constant_-1_d448d : Constant  Value=-1
  Constant_-1_dae21 : Constant  Value=-1
  Constant_-1_fc8a8 : Constant  Value=-1
  Constant_-2.0_cd8d5 : Constant  Value=-2.0
  Constant_2.0_4774e : Constant  Value=2.0
  Constant_2.0_8d880 : Constant  Value=2.0
  Constant_2.0_cea88 : Constant  Value=2.0
  Constant_D_1489d : Constant  Value=D
  Constant_H_03969 : Constant  Value=H
  Constant_f0_2c6f2 : Constant  Value=f0
  Constant_f0_8b207 : Constant  Value=f0
  Constant_f0_cfd7b : Constant  Value=f0
  Constant_pi_31251 : Constant  Value=pi
  Constant_pi_3c632 : Constant  Value=pi
  Constant_pi_f636a : Constant  Value=pi
  Constant_x_dd_55596 : Constant  Value=x_dd
  Constant_x_dd_9b69b : Constant  Value=x_dd
  Constant_x_dd_ee50a : Constant  Value=x_dd
  Constant_x_ddd_0286a : Constant  Value=x_ddd
  Constant_x_ddd_d4cb7 : Constant  Value=x_ddd
  Constant_x_ddd_ff770 : Constant  Value=x_ddd
  Constant_x_l_503e2 : Constant  Value=x_l
  Constant_x_l_53cf8 : Constant  Value=x_l
  Constant_x_l_5f5bd : Constant  Value=x_l
  Constant_x_l_77e4c : Constant  Value=x_l
  Constant_x_l_b56e6 : Constant  Value=x_l
  Constant_x_l_cf0d4 : Constant  Value=x_l
  Constant_x_qd_3b874 : Constant  Value=x_qd
  Constant_x_qd_be5ca : Constant  Value=x_qd
  Constant_x_qd_e7820 : Constant  Value=x_qd
  Constant_x_qdd_01a76 : Constant  Value=x_qdd
  Constant_x_qdd_a937c : Constant  Value=x_qdd
  Constant_x_qdd_c0335 : Constant  Value=x_qdd
  Divide_01273 : Product  Inputs=*/
  Divide_2a9c2 : Product  Inputs=*/
  Divide_66212 : Product  Inputs=*/
  Divide_7899c : Product  Inputs=*/
  Divide_8a4f7 : Product  Inputs=*/
  Divide_a980e : Product  Inputs=*/
  Divide_eb19b : Product  Inputs=*/
  Product_08cdf : Product
  Product_0e667 : Product
  Product_1b652 : Product
  Product_27f36 : Product
  Product_33f12 : Product
  Product_39792 : Product
  Product_3b020 : Product
  Product_4f811 : Product
  Product_5a6a1 : Product
  Product_5dec6 : Product
  Product_62999 : Product
  Product_a0fda : Product
  Product_a3acf : Product
  Product_a853f : Product
  Product_ad371 : Product
  Product_bcda5 : Product
  Product_c4b87 : Product
  Product_c85ae : Product
  Product_dddb5 : Product
  Product_de45e : Product
  Product_e3653 : Product
  Product_fccef : Product
  Subtract_084ce : Sum  Inputs=+-
  Subtract_1d1d5 : Sum  Inputs=+-
  Subtract_6374b : Sum  Inputs=+-
  Subtract_64d13 : Sum  Inputs=+-
  Subtract_a259c : Sum  Inputs=+-
  Subtract_a3b60 : Sum  Inputs=+-
  Subtract_a64d7 : Sum  Inputs=+-
  Subtract_cc222 : Sum  Inputs=+-
  Blockout_d_w_SG_D_3_1b2eb : Outport
  wires:
  Constant_x_qd_3b874/1 -> Subtract_1d1d5/1
  Subtract_a3b60/1 -> Product_5a6a1/2
  Subtract_6374b/1 -> Divide_66212/1
  Constant_-1_d448d/1 -> Product_3b020/1
  Add_b2220/1 -> Product_a853f/2
  Constant_x_qdd_01a76/1 -> Subtract_1d1d5/2
  Subtract_64d13/1 -> Product_39792/2
  Constant_x_l_77e4c/1 -> Product_3b020/2
  State_psi_d_SG_D_3_7b9ed/1 -> Add_0ab73/2
  Add_17440/1 -> Divide_eb19b/2
  Constant_x_dd_ee50a/1 -> Subtract_a259c/1
  Constant_x_l_cf0d4/1 -> Product_c85ae/2
  Constant_-1_fc8a8/1 -> Product_27f36/1
  Divide_8a4f7/1 -> Subtract_cc222/2
  Constant_x_ddd_ff770/1 -> Subtract_a3b60/2
  Constant_x_qdd_a937c/1 -> Add_b2220/2
  Constant_pi_3c632/1 -> Product_de45e/2
  Product_3b020/1 -> Add_b2220/1
  Constant_-2.0_cd8d5/1 -> Product_bcda5/1
  Constant_-1_4fde3/1 -> Product_c85ae/1
  Constant_2.0_8d880/1 -> Product_62999/1
  Product_bcda5/1 -> Product_a0fda/1
  Constant_-1_d0a70/1 -> Product_fccef/1
  Subtract_084ce/1 -> Add_546ba/1
  Constant_x_l_53cf8/1 -> Product_fccef/2
  Constant_x_l_5f5bd/1 -> Subtract_64d13/2
  Constant_-1_dae21/1 -> Product_0e667/1
  State_psi_1d_SG_D_3_8c18d/1 -> Product_0e667/2
  Constant_x_dd_9b69b/1 -> Subtract_a3b60/1
  Product_0e667/1 -> Product_5a6a1/1
  State_psi_gq_SG_D_3_6c331/1 -> Product_a853f/1
  Constant_x_qd_be5ca/1 -> Add_17440/2
  Product_c85ae/1 -> Add_17440/1
  State_psi_kq_SG_D_3_3748c/1 -> Product_5dec6/1
  Subtract_1d1d5/1 -> Product_5dec6/2
  Product_62999/1 -> Product_dddb5/1
  Product_a0fda/1 -> Add_0cb37/1
  Product_fccef/1 -> Add_d6f53/1
  State_psi_q_SG_D_3_3cf4a/1 -> Product_4f811/1
  Constant_x_qd_e7820/1 -> Add_d6f53/2
  Constant_x_l_503e2/1 -> Subtract_a259c/2
  Constant_x_ddd_d4cb7/1 -> Subtract_64d13/1
  Constant_x_l_b56e6/1 -> Subtract_a64d7/2
  Product_a853f/1 -> Divide_eb19b/1
  Product_5dec6/1 -> Divide_2a9c2/1
  Add_d6f53/1 -> Divide_2a9c2/2
  Product_5a6a1/1 -> Divide_01273/1
  Subtract_a259c/1 -> Divide_01273/2
  Constant_2.0_cea88/1 -> Product_de45e/1
  State_psi_fd_SG_D_3_99c58/1 -> Product_39792/1
  Constant_x_dd_55596/1 -> Subtract_a64d7/1
  Divide_eb19b/1 -> Subtract_084ce/1
  Product_39792/1 -> Divide_8a4f7/1
  Divide_2a9c2/1 -> Subtract_084ce/2
  Divide_01273/1 -> Add_0ab73/1
  Product_1b652/1 -> Subtract_6374b/2
  Subtract_a64d7/1 -> Divide_8a4f7/2
  Constant_pi_31251/1 -> Product_bcda5/2
  Constant_pi_f636a/1 -> Product_62999/2
  Constant_-1_7bc04/1 -> Product_08cdf/1
  State_psi_d_SG_D_3_3a32b/1 -> Product_08cdf/2
  State_psi_q_SG_D_3_be05f/1 -> Add_546ba/2
  Add_0ab73/1 -> Subtract_cc222/1
  Constant_f0_2c6f2/1 -> Product_a0fda/2
  Product_08cdf/1 -> Product_c4b87/1
  Add_546ba/1 -> Product_c4b87/2
  Subtract_cc222/1 -> Product_4f811/2
  Constant_D_1489d/1 -> Product_27f36/2
  State_w_SG_D_3_97bb8/1 -> Add_0cb37/2
  Product_de45e/1 -> Product_e3653/1
  State_T_m_SG_D_3_94420/1 -> Product_e3653/2
  Product_c4b87/1 -> Divide_7899c/1
  Constant_x_qdd_c0335/1 -> Divide_7899c/2
  Product_4f811/1 -> Divide_a980e/1
  Constant_x_ddd_0286a/1 -> Divide_a980e/2
  Product_27f36/1 -> Product_a3acf/1
  Add_0cb37/1 -> Product_a3acf/2
  Product_e3653/1 -> Product_33f12/1
  Constant_f0_cfd7b/1 -> Product_33f12/2
  Constant_f0_8b207/1 -> Product_dddb5/2
  Divide_7899c/1 -> Add_bd809/1
  Divide_a980e/1 -> Add_bd809/2
  Product_a3acf/1 -> Add_e8eb7/1
  Product_33f12/1 -> Add_e8eb7/2
  Product_dddb5/1 -> Product_1b652/1
  Add_bd809/1 -> Product_1b652/2
  Add_e8eb7/1 -> Subtract_6374b/1
  Constant_2.0_4774e/1 -> Product_ad371/1
  Constant_H_03969/1 -> Product_ad371/2
  Product_ad371/1 -> Divide_66212/2
  Divide_66212/1 -> Blockout_d_w_SG_D_3_1b2eb/1

== system case2/SG_D_3/i_d_SG_D_3_block ==
  note: i_d_SG_D_3 in case2
      | $\frac{\sin\left(\theta _{\mathrm{SG},D,3}\right)\,\left(\frac{\psi _{\mathrm{1d},\mathrm{SG},D,3}\,\left(x_{\mathrm{dd}}-x_{\mathrm{ddd}}\right)}{x_{\mathrm{dd}}-x_{l}}-\psi _{d,\mathrm{SG},D,3}+\frac{\psi _{\mathrm{fd},\mathrm{SG},D,3}\,\left(x_{\mathrm{ddd}}-x_{l}\right)}{x_{\mathrm{dd}}-x_{l}}\right)}{x_{\mathrm{ddd}}}-\frac{\cos\left(\theta _{\mathrm{SG},D,3}\right)\,\left(\psi _{q,\mathrm{SG},D,3}+\frac{\psi _{\mathrm{gq},\mathrm{SG},D,3}\,\left(x_{l}-x_{\mathrm{qdd}}\right)}{x_{l}-x_{\mathrm{qd}}}+\frac{\psi _{\mathrm{kq},\mathrm{SG},D,3}\,\left(x_{\mathrm{qd}}-x_{\mathrm{qdd}}\right)}{x_{l}-x_{\mathrm{qd}}}\right)}{x_{\mathrm{qdd}}}$
      | Automatically generated on 2025-10-31 18:56:13 .
  State_psi_gq_SG_D_3_d77e8 : Inport
  State_psi_kq_SG_D_3_36d89 : Inport  Port=2
  State_psi_q_SG_D_3_0448a : Inport  Port=3
  State_theta_SG_D_3_a77c5 : Inport  Port=4
  State_psi_1d_SG_D_3_0bb66 : Inport  Port=5
  State_psi_d_SG_D_3_23dc4 : Inport  Port=6
  State_psi_fd_SG_D_3_d8144 : Inport  Port=7
  State_theta_SG_D_3_da351 : Inport  Port=8
  Add_23733 : Sum
  Add_501d5 : Sum
  Add_c2669 : Sum
  Add_e07ec : Sum
  Add_f311e : Sum
  Constant_-1_5befe : Constant  Value=-1
  Constant_-1_87c84 : Constant  Value=-1
  Constant_-1_9b0ad : Constant  Value=-1
  Constant_-1_9bc7c : Constant  Value=-1
  Constant_-1_e39e9 : Constant  Value=-1
  Constant_x_dd_0dfc7 : Constant  Value=x_dd
  Constant_x_dd_8d661 : Constant  Value=x_dd
  Constant_x_dd_91077 : Constant  Value=x_dd
  Constant_x_ddd_43e7b : Constant  Value=x_ddd
  Constant_x_ddd_8efaa : Constant  Value=x_ddd
  Constant_x_ddd_94a49 : Constant  Value=x_ddd
  Constant_x_l_23770 : Constant  Value=x_l
  Constant_x_l_3b3b0 : Constant  Value=x_l
  Constant_x_l_48248 : Constant  Value=x_l
  Constant_x_l_da6a6 : Constant  Value=x_l
  Constant_x_l_efeac : Constant  Value=x_l
  Constant_x_l_fff8d : Constant  Value=x_l
  Constant_x_qd_661e3 : Constant  Value=x_qd
  Constant_x_qd_9b5d2 : Constant  Value=x_qd
  Constant_x_qd_db733 : Constant  Value=x_qd
  Constant_x_qdd_7ae84 : Constant  Value=x_qdd
  Constant_x_qdd_84a75 : Constant  Value=x_qdd
  Constant_x_qdd_a2292 : Constant  Value=x_qdd
  Divide_1c190 : Product  Inputs=*/
  Divide_43f51 : Product  Inputs=*/
  Divide_68cdc : Product  Inputs=*/
  Divide_c3089 : Product  Inputs=*/
  Divide_c4cd6 : Product  Inputs=*/
  Divide_ff5b4 : Product  Inputs=*/
  MathFunc_cos_49500 : Trigonometry  Operator=cos
  MathFunc_sin_a6731 : Trigonometry
  Product_01fad : Product
  Product_080fd : Product
  Product_3e9c7 : Product
  Product_72990 : Product
  Product_7a68b : Product
  Product_86e6a : Product
  Product_a52cd : Product
  Product_bef42 : Product
  Product_c4abb : Product
  Product_d2701 : Product
  Product_e995a : Product
  Subtract_19d6f : Sum  Inputs=+-
  Subtract_1ce10 : Sum  Inputs=+-
  Subtract_3ad27 : Sum  Inputs=+-
  Subtract_413cc : Sum  Inputs=+-
  Subtract_59dc3 : Sum  Inputs=+-
  Subtract_6235e : Sum  Inputs=+-
  Subtract_eaf4c : Sum  Inputs=+-
  Subtract_fad70 : Sum  Inputs=+-
  Blockout_i_d_SG_D_3_0a1a0 : Outport
  wires:
  Constant_x_qd_661e3/1 -> Subtract_413cc/1
  Subtract_3ad27/1 -> Blockout_i_d_SG_D_3_0a1a0/1
  Constant_-1_5befe/1 -> Product_01fad/1
  Constant_x_l_efeac/1 -> Product_7a68b/2
  Constant_x_qdd_84a75/1 -> Add_501d5/2
  Constant_x_qdd_a2292/1 -> Subtract_413cc/2
  Constant_x_l_da6a6/1 -> Product_01fad/2
  Divide_ff5b4/1 -> Subtract_3ad27/1
  Product_01fad/1 -> Add_501d5/1
  Constant_x_ddd_43e7b/1 -> Subtract_1ce10/2
  Constant_-1_9bc7c/1 -> Product_7a68b/1
  Constant_-1_e39e9/1 -> Product_a52cd/1
  Constant_x_l_48248/1 -> Product_a52cd/2
  State_psi_1d_SG_D_3_0bb66/1 -> Product_72990/2
  State_psi_gq_SG_D_3_d77e8/1 -> Product_86e6a/1
  Product_72990/1 -> Product_e995a/1
  Add_501d5/1 -> Product_86e6a/2
  Product_7a68b/1 -> Add_f311e/1
  Constant_x_qd_db733/1 -> Add_f311e/2
  State_psi_kq_SG_D_3_36d89/1 -> Product_c4abb/1
  Subtract_6235e/1 -> Divide_1c190/2
  Subtract_413cc/1 -> Product_c4abb/2
  Product_a52cd/1 -> Add_23733/1
  Constant_x_ddd_94a49/1 -> Subtract_fad70/1
  Constant_x_qd_9b5d2/1 -> Add_23733/2
  Constant_-1_87c84/1 -> Product_72990/1
  Constant_x_dd_91077/1 -> Subtract_1ce10/1
  Product_86e6a/1 -> Divide_43f51/1
  Add_f311e/1 -> Divide_43f51/2
  Product_c4abb/1 -> Divide_68cdc/1
  Add_23733/1 -> Divide_68cdc/2
  Divide_1c190/1 -> Subtract_59dc3/2
  Subtract_1ce10/1 -> Product_e995a/2
  State_theta_SG_D_3_a77c5/1 -> MathFunc_cos_49500/1
  Constant_x_dd_8d661/1 -> Subtract_eaf4c/1
  Product_bef42/1 -> Product_d2701/1
  Constant_x_l_fff8d/1 -> Subtract_eaf4c/2
  Add_e07ec/1 -> Subtract_59dc3/1
  Constant_x_l_3b3b0/1 -> Subtract_fad70/2
  State_theta_SG_D_3_da351/1 -> MathFunc_sin_a6731/1
  Divide_43f51/1 -> Subtract_19d6f/1
  Add_c2669/1 -> Product_bef42/2
  Divide_68cdc/1 -> Subtract_19d6f/2
  Product_e995a/1 -> Divide_c3089/1
  Subtract_eaf4c/1 -> Divide_c3089/2
  State_psi_fd_SG_D_3_d8144/1 -> Product_3e9c7/1
  Divide_c4cd6/1 -> Subtract_3ad27/2
  Subtract_fad70/1 -> Product_3e9c7/2
  Constant_x_dd_0dfc7/1 -> Subtract_6235e/1
  Subtract_19d6f/1 -> Add_c2669/1
  Constant_x_l_23770/1 -> Subtract_6235e/2
  Constant_-1_9b0ad/1 -> Product_bef42/1
  State_psi_q_SG_D_3_0448a/1 -> Add_c2669/2
  Divide_c3089/1 -> Add_e07ec/1
  State_psi_d_SG_D_3_23dc4/1 -> Add_e07ec/2
  Product_3e9c7/1 -> Divide_1c190/1
  MathFunc_cos_49500/1 -> Product_d2701/2
  MathFunc_sin_a6731/1 -> Product_080fd/2
  Subtract_59dc3/1 -> Product_080fd/1
  Product_d2701/1 -> Divide_ff5b4/1
  Constant_x_qdd_7ae84/1 -> Divide_ff5b4/2
  Product_080fd/1 -> Divide_c4cd6/1
  Constant_x_ddd_8efaa/1 -> Divide_c4cd6/2
